simulink model "modi1_7"  (R2022b)
settings: Solver=VariableStepAuto  StartTime=0.0  StopTime=100.0  RelTol=1e-3
values from neighbouring files (symbols this model uses):
  a0 = 0.00447127    [modi1.m]
  a1 = 0.108205    [modi1.m]
  a2 = 0.683702    [modi1.m]
  alfa1 = 1.2    [modi1.m]
  alfa2 = 0.56    [modi1.m]
  alfa3 = -1.45    [modi1.m]
  alfa4 = 1.15    [modi1.m]
  b0 = 0.00201207    [modi1.m]
  T = 2.5    [modi1.m]
settings Model: Creator=zalew  LastModifiedBy=zalew

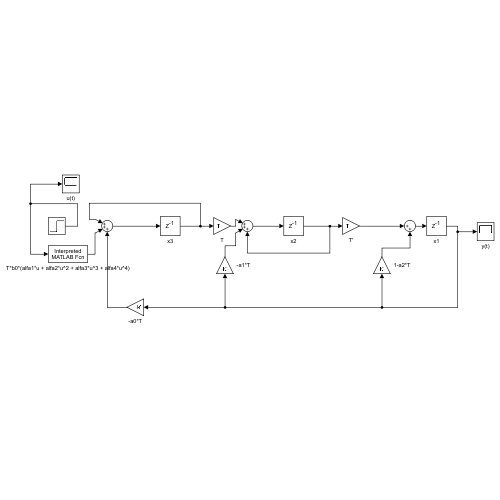
[thumbnail: Simulink's stored preview of the top-level diagram]
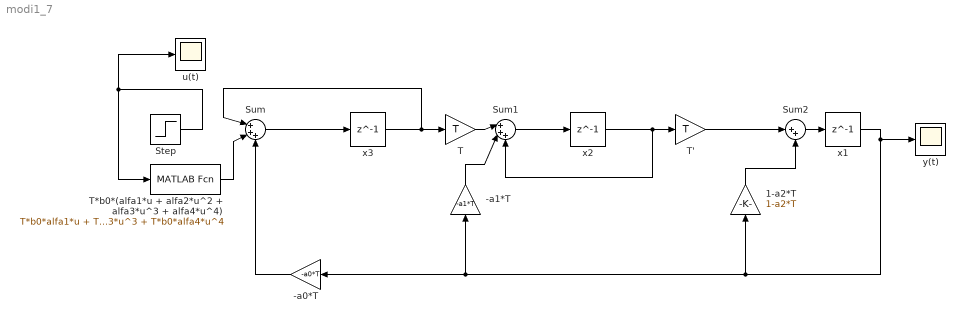
== system modi1_7 ==
  -a0*T : Gain  Gain=-a0*T
  -a1*T : Gain  Gain=-a1*T
  1-a2*T : Gain  Gain=1-a2*T
  Step : Step  Time=10  After=0.5  SampleTime=0
  Sum : Sum  Inputs=|+++
  Sum1 : Sum  Inputs=|+++
  Sum2 : Sum  Inputs=|++
  T : Gain  Gain=T
  T' : Gain  Gain=T
  T*b0*(alfa1*u + alfa2*u^2 + alfa3*u^3 + alfa4*u^4) : MATLABFcn  MATLABFcn=T*b0*alfa1*u + T*b0*alfa2*u^2 + T*b0*alfa3*u^3 + T*b0*alfa4*u^4
  u(t) : Scope
  x1 : Delay  DelayLength=1  InitialCondition=0  SampleTime=T
  x2 : Delay  DelayLength=1  InitialCondition=0  SampleTime=T
  x3 : Delay  DelayLength=1  InitialCondition=0  SampleTime=T
  y(t) : Scope
  wires:
  Sum/1 -> x3/1
  x3/1 -> Sum/1, T/1
  T*b0*(alfa1*u + alfa2*u^2 + alfa3*u^3 + alfa4*u^4)/1 -> Sum/2
  x1/1 -> -a0*T/1, -a1*T/1, 1-a2*T/1, y(t)/1
  -a0*T/1 -> Sum/3
  T/1 -> Sum1/1
  -a1*T/1 -> Sum1/2
  x2/1 -> T'/1, Sum1/3
  Sum1/1 -> x2/1
  T'/1 -> Sum2/1
  1-a2*T/1 -> Sum2/2
  Sum2/1 -> x1/1
  Step/1 -> u(t)/1, T*b0*(alfa1*u + alfa2*u^2 + alfa3*u^3 + alfa4*u^4)/1
